simulink model "psbcontrolcurr"  (Simulink 6.0)
settings: Solver=VariableStepDiscrete  SolverMode=SingleTasking  StartTime=0.0  StopTime=100  MaxStep=1e-03  RelTol=1e-3  AbsTol=1e-6
libraries: powerlib2 x5
settings Model: Creator=patrice  LastModifiedBy=batserve  ExtModeTrigMode=oneshot  ExtModeArmWhenConnect=off  ExtModeAutoUpdateStatusClock=off
settings DataIOCC: LimitDataPoints=off  SignalLoggingName=sigsOut
settings OptimizationCC: BooleanDataType=off
settings DebuggingCC: SolverPrmCheckMsg=none
settings HardwareCC: TargetUnknown=on
settings RTWCC: TemplateMakefile=grt_unix.tmf

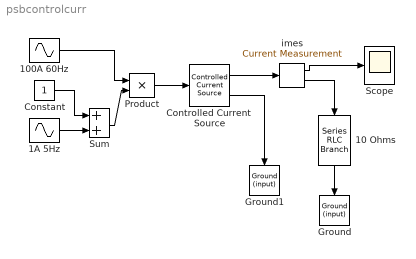
== system psbcontrolcurr ==
  "10 Ohms " : powerlib2/Elements/Series RLC Branch  Tag=PoWeRsYsTeMbLoCk  Orientation=down  a=10  b=0  c=inf  mesure=None  PSBOutputType=1
  100A 60Hz : Sin  Amplitude=100  Frequency=2*pi*60  SampleTime=0
  1A 5Hz : Sin  Frequency=2*pi*5  SampleTime=0
  Constant : Constant
  Controlled Current  Source : powerlib2/Electrical Sources/Controlled Current Source  Tag=PoWeRsYsTeMbLoCk  initsrc=on  srctyp=AC  ia=0  iph=0  freq=0  mesure=None  PSBOutputType=11
  Ground : powerlib2/Connectors/Ground (input)  Tag=PoWeRsYsTeMbLoCk  Orientation=down
  Ground1 : powerlib2/Connectors/Ground (input)  Tag=PoWeRsYsTeMbLoCk  Orientation=down
  Product : Product  SaturateOnIntegerOverflow=on  InputSameDT=on
  Scope : Scope
      settings: TickLabels=on  TimeRange=0.5  YMin=-200  YMax=200  DataFormat=Array
  Sum : Sum  SaturateOnIntegerOverflow=on  InputSameDT=on
  imes : powerlib2/Measurements/Current Measurement  Tag=PoWeRsYsTeMmEaSuReMeNt  PhasorSimulation=off  OutputType=Magnitude  PSBOutputType=01  PSBequivalent=0
  wires:
  "10 Ohms "/1 -> Ground/1
  imes/2 -> "10 Ohms "/1
  imes/1 -> Scope/1
  1A 5Hz/1 -> Sum/2
  Controlled Current  Source/2 -> Ground1/1
  Controlled Current  Source/1 -> imes/1
  Product/1 -> Controlled Current  Source/1
  Constant/1 -> Sum/1
  Sum/1 -> Product/2
  100A 60Hz/1 -> Product/1
